simulink model "delay_block"  (R2022b)
settings: Solver=VariableStepAuto  StartTime=0.0  StopTime=100  RelTol=1e-3
settings Model: Creator=alexg  LastModifiedBy=alexg

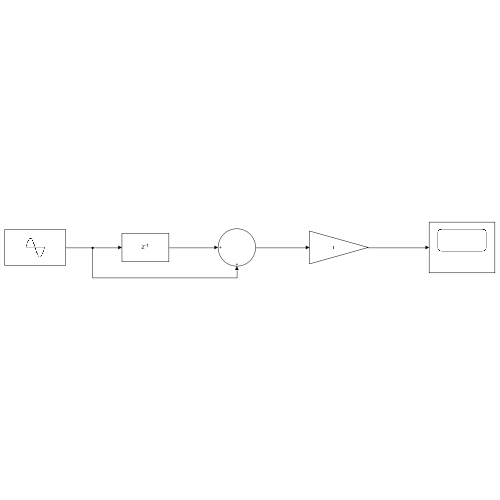
[thumbnail: Simulink's stored preview of the top-level diagram]
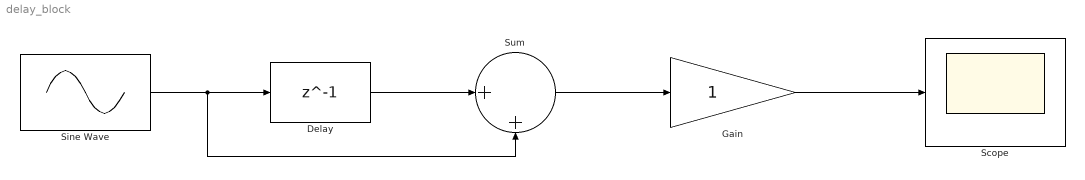
== system delay_block ==
  Delay : Delay  DelayLength=1  InitialCondition=0
  Gain : Gain
  Scope : Scope
  Sine Wave : Sin  SampleTime=0
  Sum : Sum  Inputs=|++
  wires:
  Delay/1 -> Sum/1
  Sine Wave/1 -> Sum/2, Delay/1
  Sum/1 -> Gain/1
  Gain/1 -> Scope/1
